simulink model "RpiFinalLEDLong"  (R2023a)
settings: Solver=FixedStepDiscrete  StartTime=0.0  StopTime=48  RelTol=1e-3  EnableMultiTasking=on
undefined symbols (not defined in the file): Green, led0
libraries: embmathops x2, simulink x1, raspberrypiBasiclib x1
settings Model: ModifiedByFormat=The MathWorks Inc.  SimulationMode=external  ExtModeTrigDuration=2  Creator=The MathWorks, Inc.  LastModifiedBy=The MathWorks Inc.
settings SolverCC: AlgebraicLoopSolver=TrustRegion  PositivePriorityOrder=on  AutoInsertRateTranBlk=on  MaxZcPerStep=1
settings DataIOCC: LimitDataPoints=on  SaveFormat=Array  ReturnWorkspaceOutputs=off
settings OptimizationCC: ReuseModelBlockBuffer=off  LifeSpan=1  MaxStackSize=64
settings DebuggingCC: UnderspecifiedInitializationDetection=Classic  MergeDetectMultiDrivingBlocksExec=none  SolverPrmCheckMsg=warning  UnconnectedInputMsg=warning  UnconnectedOutputMsg=warning  UnconnectedLineMsg=warning  AllowSymbolicDim=off  SFUnexpectedBacktrackingDiag=warning  SFNoUnconditionalDefaultTransitionDiag=warning  SFExecutionAtInitializationDiag=none  ArithmeticOperatorsInVariantConditions=warning
settings HardwareCC: ProdBitPerPointer=32  ProdBitPerSizeT=32  ProdBitPerPtrDiffT=32  ProdLargestAtomicInteger=Long  ProdLargestAtomicFloat=Double  ProdWordSize=32  ProdHWDeviceType=ARM Compatible->ARM Cortex  UseEmbeddedCoderFeatures=off  UseSimulinkCoderFeatures=off
settings ModelReferenceCC: EnableRefExpFcnMdlSchedulingChecks=on  PropagateSignalLabelsOutOfModel=off
settings SFSimCC: SimUseLocalCustomCode=off  MATLABDynamicMemAlloc=off  CustomCodeUndefinedFunction=UseInterfaceOnly
settings RTWCC: Description=Embedded Coder  SystemTargetFile=ert.tlc  HardwareBoard=Raspberry Pi  TemplateMakefile=ert_default_tmf  RTWUseLocalCustomCode=off  Toolchain=GNU GCC Embedded Linux  DLArmComputeVersion=19.05
settings CodeAppCC: MangleLength=10  StateflowObjectComments=on
settings ERTTargetCC: MultiwordLength=2048  ERTCustomFileBanners=off  SupportContinuousTime=on  SupportNonInlinedSFcns=on  RemoveResetFunc=off  ModelStepFunctionPrototypeControlCompliant=off  ConvertIfToSwitch=off  SuppressUnreachableDefaultCases=off
settings ConfigComp: CovMetricSettings=dw  CovSaveCumulativeToWorkspaceVar=on  CovSaveSingleToWorkspaceVar=on  CovExternalEMLEnable=off  CovSFcnEnable=off

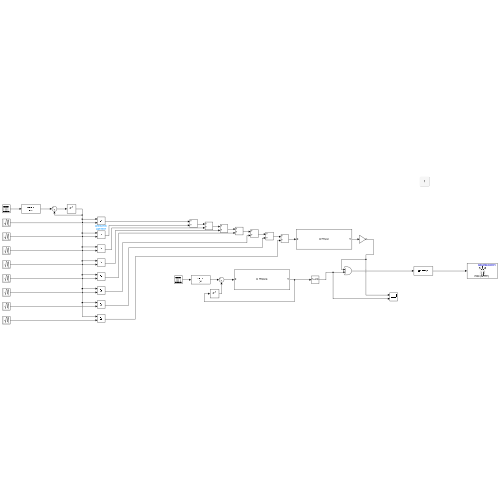
[thumbnail: Simulink's stored preview of the top-level diagram]
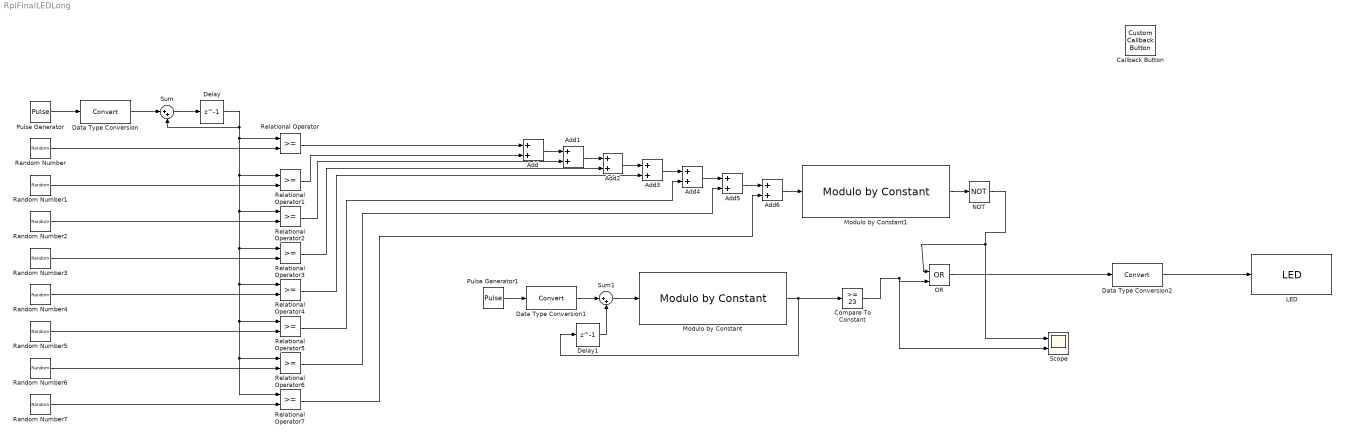
== system RpiFinalLEDLong ==
  Add{,1..6} (7 alike) : Sum
  Callback Button : CustomCallbackButton  Configuration="{\"components\":[{\"name\":\"BackgroundImageComponent\",\"settings\":{\"image\":{\"size\":[0,0],\"src\":\"default\",\"srcOrientation\":\"Right\"},\"position\":[0,0,1,1]}},{\"name\":\"ButtonStateComponent\",\"settings\":{\"buttonType\":\"momentary\",\"clickFcn\":\"showExample('raspberrypi\\/GettingStartedWithSimulinkRaspberryPiHardwareExample')\",\"onValue\":1,\"position\":[0,0,1,1],\"pressDelay\":\"500\",\"pressFcn\":\"\",\"repeatInterval\":\"0\",\"states\":[{\"horizontalAlignment\":\"center\",\"image\":{\"position\":[0,0,1,1],\"src\":\"default\",\"srcOrientation\":\"Right\"},\"label\":{\"color\":[0.01176470588,0.01176470588,0.01176470588,1],\"icon\":{\"size\":[0,0],\"src\":\"default\",\"srcOrientation\":\"Right\"},\"iconPlacement\":\"left\",\"text\":{\"content\":\"?\"}},\"labelOffset\":[0,0],\"verticalAlignment\":\"middle\"},{\"horizontalAlignment\":\"center\",\"image\":{\"position\":[0,0,1,1],\"src\":\"default\",\"srcOrientation\":\"Right\"},\"label\":{\"color\":[0.01176470588,0.01176470588,0.01176470588,1],\"icon\":{\"size\":[0,0],\"src\":\"default\",\"srcOrientation\":\"Right\"},\"iconPlacement\":\"left\",\"text\":{\"content\":\"?\"}},\"labelOffset\":[0,0],\"verticalAlignment\":\"middle\"},{\"horizontalAlignment\":\"center\",\"image\":{\"position\":[0,0,1,1],\"src\":\"default\",\"srcOrientation\":\"Right\"},\"label\":{\"color\":[0.01176470588,0.01176470588,0.01176470588,1],\"icon\":{\"size\":[0,0],\"src\":\"default\",\"srcOrientation\":\"Right\"},\"iconPlacement\":\"left\",\"text\":{\"content\":\"?\"}},\"labelOffset\":[0,0],\"verticalAlignment\":\"middle\"},{\"horizontalAlignment\":\"center\",\"image\":{\"position\":[0,0,1,1],\"src\":\"default\",\"srcOrientation\":\"Right\"},\"label\":{\"color\":[0.01176470588,0.01176470588,0.01176470588,1],\"icon\":{\"size\":[0,0],\"src\":\"default\",\"srcOrientation\":\"Right\"},\"iconPlacement\":\"left\",\"text\":{\"content\":\"?\"}},\"labelOffset\":[0,0],\"verticalAlignment\":\"middle\"}]}},{\"name\":\"ForegroundImageComponent\",\"settings\":{\"image\":{\"size\":[0,0],\"src\":\"default\",\"srcOrientation\":\"Right\"},\"isForeground\":1,\"position\":[0,0,1,1]}}],\"settings\":{\"BindingType\":\"standalone\",\"backgroundColor\":[244,244,244,1],\"backgroundOffset\":0.2,\"backgroundOpacity\":1,\"fixedAspectRatio\":\"off\",\"foregroundColor\":[0.01176470588,0.01176470588,0.01176470588,1],\"migratedFromLegacy\":true,\"useBackgroundColor\":true,\"variant\":\"callback\",\"version\":\"R2023a\"},\"type\":\"Button\"}"  CustomBackgroundColor="{\"color\":[0.9568627450980393,0.9568627450980393,0.9568627450980393],\"show\":true}"
  Compare To Constant : simulink/Logic and Bit Operations/Compare To Constant  relop=>=  const=23  OutDataTypeStr=boolean
  Data Type Conversion : DataTypeConversion  OutMin=0  OutMax=1  ConvertRealWorld=Stored Integer (SI)  RndMeth=Nearest  SaturateOnIntegerOverflow=off
  Data Type Conversion1 : DataTypeConversion  OutMin=0  OutMax=1  ConvertRealWorld=Stored Integer (SI)  RndMeth=Nearest  SaturateOnIntegerOverflow=off
  Data Type Conversion2 : DataTypeConversion  SaturateOnIntegerOverflow=off  RndMeth=Floor
  Delay : Delay  DelayLength=1  InitialCondition=0  SampleTime=1
  Delay1 : Delay  DelayLength=1  InitialCondition=0  SampleTime=1
  LED : raspberrypiBasiclib/LED  BoardProperty=Pi 3 Model B+  LED_=led0 (Green)
  Modulo by Constant : embmathops/Modulo by Constant  Denominator=24  SimulateUsing=Code generation
      settings: LibrarySourceBlock=embeddedMathLib/Modulo by Constant
  Modulo by Constant1 : embmathops/Modulo by Constant  Denominator=2  SimulateUsing=Code generation
      settings: LibrarySourceBlock=embeddedMathLib/Modulo by Constant
  NOT : Logic  Operator=NOT  IconShape=distinctive  AllPortsSameDT=off  OutDataTypeStr=boolean
  OR : Logic  Operator=OR  IconShape=distinctive  AllPortsSameDT=off  OutDataTypeStr=boolean
  Pulse Generator : DiscretePulseGenerator  Period=1  SampleTime=48
  Pulse Generator1 : DiscretePulseGenerator  Period=10  PulseWidth=5
  Random Number : RandomNumber  Mean=3  SampleTime=48
  Random Number1 : RandomNumber  Mean=9  Seed=1  SampleTime=48
  Random Number2 : RandomNumber  Mean=15  Seed=2  SampleTime=48
  Random Number3 : RandomNumber  Mean=21  Seed=3  SampleTime=48
  Random Number4 : RandomNumber  Mean=27  Seed=4  SampleTime=48
  Random Number5 : RandomNumber  Mean=33  Seed=5  SampleTime=48
  Random Number6 : RandomNumber  Mean=39  Seed=6  SampleTime=48
  Random Number7 : RandomNumber  Mean=45  Seed=7  SampleTime=48
  Relational Operator{,1..7} (8 alike) : RelationalOperator  OutDataTypeStr=boolean  RndMeth=Simplest  InputSameDT=off
  Scope : Scope  NumInputPorts=2
  Sum : Sum  Inputs=|++
  Sum1 : Sum  Inputs=|++
  wires:
  OR/1 -> Data Type Conversion2/1
  Modulo by Constant/1 -> Compare To Constant/1, Delay1/1
  Compare To Constant/1 -> Scope/2, OR/2
  Delay1/1 -> Sum1/2
  Data Type Conversion1/1 -> Sum1/1
  Pulse Generator1/1 -> Data Type Conversion1/1
  Sum1/1 -> Modulo by Constant/1
  NOT/1 -> Scope/1, OR/1
  Data Type Conversion2/1 -> LED/1
  Random Number2/1 -> Relational Operator2/2
  Relational Operator6/1 -> Add5/2
  Relational Operator4/1 -> Add3/2
  Random Number3/1 -> Relational Operator3/2
  Random Number/1 -> Relational Operator/2
  Relational Operator2/1 -> Add1/2
  Random Number6/1 -> Relational Operator6/2
  Relational Operator5/1 -> Add4/2
  Relational Operator3/1 -> Add2/2
  Delay/1 -> Relational Operator/1, Relational Operator6/1, Relational Operator7/1, Relational Operator5/1, Relational Operator4/1, Relational Operator3/1, Relational Operator2/1, Relational Operator1/1, Sum/2
  Add3/1 -> Add4/1
  Relational Operator1/1 -> Add/2
  Relational Operator/1 -> Add/1
  Add6/1 -> Modulo by Constant1/1
  Add/1 -> Add1/1
  Add5/1 -> Add6/1
  Add2/1 -> Add3/1
  Random Number1/1 -> Relational Operator1/2
  Add4/1 -> Add5/1
  Data Type Conversion/1 -> Sum/1
  Modulo by Constant1/1 -> NOT/1
  Random Number5/1 -> Relational Operator5/2
  Add1/1 -> Add2/1
  Relational Operator7/1 -> Add6/2
  Random Number7/1 -> Relational Operator7/2
  Random Number4/1 -> Relational Operator4/2
  Pulse Generator/1 -> Data Type Conversion/1
  Sum/1 -> Delay/1
